simulink model "testMaxonMotors"  (R2013b)
settings: Solver=VariableStepDiscrete  StartTime=0.0  StopTime=65  RelTol=1e-3
settings Model: Creator=eugenio  LastModifiedBy=eyime
settings DataIOCC: SignalLoggingSaveFormat=ModelDataLogs
settings OptimizationCC: ExpressionDepthLimit=2147483647
settings DebuggingCC: FcnCallInpInsideContextMsg=UseLocalSettings  StateNameClashWarn=warning
settings SFSimCC: SimParseCustomCode=off
settings GRTTargetCC: CombineOutputUpdateFcns=off  GRTInterface=on
settings SimMechanicsCC: VisDuringSimulation=on
settings ConfigurationSet: Description=SimMechanics 2G

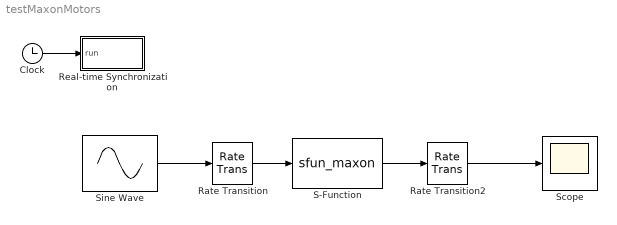
== system testMaxonMotors ==
  Clock : Clock
  Rate Transition : RateTransition
  Rate Transition2 : RateTransition
  Real-time Synchronization : Subsystem
  S-Function : S-Function  FunctionName=sfun_maxon  Parameters=NodeID, DeltaT, OpMode  EnableBusSupport=off  mask{NodeID=1, DeltaT=0.01, OpMode=3}
      mask prompts: DeltaT "Delta T"; OpMode "Operational Mode"
  Scope : Scope
      settings: YMin=-150000  YMax=150000
  Sine Wave : Sin  Amplitude=132000  Frequency=0.1  SampleTime=0
  wires:
  Rate Transition/1 -> S-Function/1
  Sine Wave/1 -> Rate Transition/1
  S-Function/1 -> Rate Transition2/1
  Rate Transition2/1 -> Scope/1
  Clock/1 -> Real-time Synchronization/1(run)

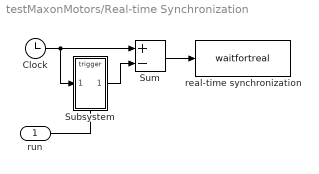
== system testMaxonMotors/Real-time Synchronization ==
  run : Inport
  Clock : Clock
  Subsystem : Subsystem  TreatAsAtomicUnit=on
  Sum : Sum  Inputs=+-  SaturateOnIntegerOverflow=on  InputSameDT=on  OutDataTypeStr=Inherit: Same as first input
  real-time synchronization : MATLABFcn  MATLABFcn=waitfortreal  OutputDimensions=0
  wires:
  Clock/1 -> Subsystem/1(In), Sum/1
  Subsystem/1(Out) -> Sum/2
  Sum/1 -> real-time synchronization/1
  run/1 -> Subsystem/Trigger

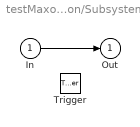
== system testMaxonMotors/Real-time Synchronization/Subsystem ==
  In : Inport
  Trigger : TriggerPort
  Out : Outport  InitialOutput=0
  wires:
  In/1 -> Out/1
